simulink model "BMS_DCDC_Manager_V1"  (R2024b)
settings: Solver=FixedStepDiscrete  StartTime=0.0  StopTime=1  FixedStep=0.1  RelTol=1e-3
settings Model: Creator=Jingjing.jiang  LastModifiedBy=Jingjing.jiang
settings DataIOCC: SaveFormat=StructureWithTime

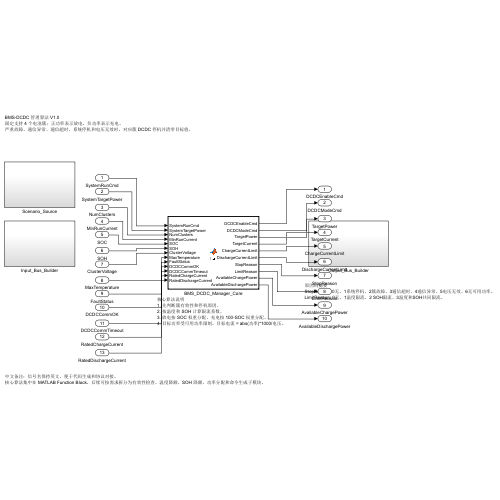
[thumbnail: Simulink's stored preview of the top-level diagram]
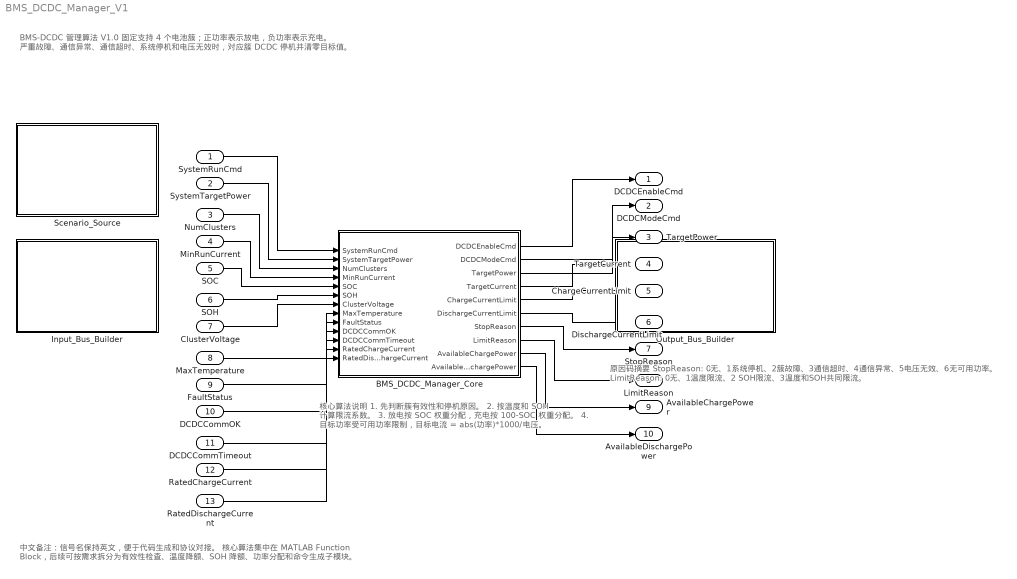
== system BMS_DCDC_Manager_V1 ==
  note: BMS-DCDC 管理算法 V1.0
      | 固定支持 4 个电池簇；正功率表示放电，负功率表示充电。
      | 严重故障、通信异常、通信超时、系统停机和电压无效时，对应簇 DCDC 停机并清零目标值。
  note: 中文备注：信号名保持英文，便于代码生成和协议对接。
      | 核心算法集中在 MATLAB Function Block，后续可按需求拆分为有效性检查、温度降额、SOH 降额、功率分配和命令生成子模块。
  note: 核心算法说明
      | 1. 先判断簇有效性和停机原因。
      | 2. 按温度和 SOH 计算限流系数。
      | 3. 放电按 SOC 权重分配，充电按 100-SOC 权重分配。
      | 4. 目标功率受可用功率限制，目标电流 = abs(功率)*1000/电压。
  note: 原因码摘要
      | StopReason: 0无、1系统停机、2簇故障、3通信超时、4通信异常、5电压无效、6无可用功率。
      | LimitReason: 0无、1温度限流、2 SOH限流、3温度和SOH共同限流。
  SystemRunCmd : Inport  OutDataTypeStr=boolean  PortDimensions=1
  SystemTargetPower : Inport  Port=2  OutDataTypeStr=double  PortDimensions=1
  NumClusters : Inport  Port=3  OutDataTypeStr=uint8  PortDimensions=1
  MinRunCurrent : Inport  Port=4  OutDataTypeStr=double  PortDimensions=1
  SOC : Inport  Port=5  OutDataTypeStr=double  PortDimensions=4
  SOH : Inport  Port=6  OutDataTypeStr=double  PortDimensions=4
  ClusterVoltage : Inport  Port=7  OutDataTypeStr=double  PortDimensions=4
  MaxTemperature : Inport  Port=8  OutDataTypeStr=double  PortDimensions=4
  FaultStatus : Inport  Port=9  OutDataTypeStr=boolean  PortDimensions=4
  DCDCCommOK : Inport  Port=10  OutDataTypeStr=boolean  PortDimensions=4
  DCDCCommTimeout : Inport  Port=11  OutDataTypeStr=boolean  PortDimensions=4
  RatedChargeCurrent : Inport  Port=12  OutDataTypeStr=double  PortDimensions=4
  RatedDischargeCurrent : Inport  Port=13  OutDataTypeStr=double  PortDimensions=4
  BMS_DCDC_Manager_Core : MATLAB Function  TreatAsAtomicUnit=on
  Input_Bus_Builder : Subsystem
  Output_Bus_Builder : Subsystem
  Scenario_Source : Subsystem
  DCDCEnableCmd : Outport  OutDataTypeStr=boolean  PortDimensions=4
  DCDCModeCmd : Outport  Port=2  OutDataTypeStr=uint8  PortDimensions=4
  TargetPower : Outport  Port=3  OutDataTypeStr=double  PortDimensions=4
  TargetCurrent : Outport  Port=4  OutDataTypeStr=double  PortDimensions=4
  ChargeCurrentLimit : Outport  Port=5  OutDataTypeStr=double  PortDimensions=4
  DischargeCurrentLimit : Outport  Port=6  OutDataTypeStr=double  PortDimensions=4
  StopReason : Outport  Port=7  OutDataTypeStr=uint16  PortDimensions=4
  LimitReason : Outport  Port=8  OutDataTypeStr=uint16  PortDimensions=4
  AvailableChargePower : Outport  Port=9  OutDataTypeStr=double  PortDimensions=4
  AvailableDischargePower : Outport  Port=10  OutDataTypeStr=double  PortDimensions=4
  wires:
  SystemRunCmd/1 -> BMS_DCDC_Manager_Core/1(SystemRunCmd)
  SystemTargetPower/1 -> BMS_DCDC_Manager_Core/2(SystemTargetPower)
  NumClusters/1 -> BMS_DCDC_Manager_Core/3(NumClusters)
  MinRunCurrent/1 -> BMS_DCDC_Manager_Core/4(MinRunCurrent)
  SOC/1 -> BMS_DCDC_Manager_Core/5(SOC)
  SOH/1 -> BMS_DCDC_Manager_Core/6(SOH)
  ClusterVoltage/1 -> BMS_DCDC_Manager_Core/7(ClusterVoltage)
  MaxTemperature/1 -> BMS_DCDC_Manager_Core/8(MaxTemperature)
  FaultStatus/1 -> BMS_DCDC_Manager_Core/9(FaultStatus)
  DCDCCommOK/1 -> BMS_DCDC_Manager_Core/10(DCDCCommOK)
  DCDCCommTimeout/1 -> BMS_DCDC_Manager_Core/11(DCDCCommTimeout)
  RatedChargeCurrent/1 -> BMS_DCDC_Manager_Core/12(RatedChargeCurrent)
  RatedDischargeCurrent/1 -> BMS_DCDC_Manager_Core/13(RatedDischargeCurrent)
  BMS_DCDC_Manager_Core/1(DCDCEnableCmd) -> DCDCEnableCmd/1
  BMS_DCDC_Manager_Core/2(DCDCModeCmd) -> DCDCModeCmd/1
  BMS_DCDC_Manager_Core/3(TargetPower) -> TargetPower/1
  BMS_DCDC_Manager_Core/4(TargetCurrent) -> TargetCurrent/1
  BMS_DCDC_Manager_Core/5(ChargeCurrentLimit) -> ChargeCurrentLimit/1
  BMS_DCDC_Manager_Core/6(DischargeCurrentLimit) -> DischargeCurrentLimit/1
  BMS_DCDC_Manager_Core/7(StopReason) -> StopReason/1
  BMS_DCDC_Manager_Core/8(LimitReason) -> LimitReason/1
  BMS_DCDC_Manager_Core/9(AvailableChargePower) -> AvailableChargePower/1
  BMS_DCDC_Manager_Core/10(AvailableDischargePower) -> AvailableDischargePower/1

== system BMS_DCDC_Manager_V1/Input_Bus_Builder ==
  note: 输入接口说明
      | 系统级输入：SystemRunCmd、SystemTargetPower、NumClusters、MinRunCurrent。
      | 簇级数组固定 4 维：SOC、SOH、电压、温度、故障、通信和额定电流。

== system BMS_DCDC_Manager_V1/Output_Bus_Builder ==
  note: 输出接口说明
      | DCDCEnableCmd：启停命令。
      | DCDCModeCmd：0=待机，1=充电，2=放电，3=故障。
      | TargetCurrent 始终为正值，方向由模式命令区分。

== system BMS_DCDC_Manager_V1/Scenario_Source ==
  note: 测试激励 / Scenario_Source
      | 默认场景数据来自 BMS_DCDC_Params.m。
      | TC01~TC08 可在自检脚本和后续测试模型中扩展。

== matlab function BMS_DCDC_Manager_V1/BMS_DCDC_Manager_Core ==
  data: SystemRunCmd input; DCDCEnableCmd output; SystemTargetPower input; NumClusters input; MinRunCurrent input; SOC input; SOH input; ClusterVoltage input; MaxTemperature input; FaultStatus input; DCDCCommOK input; DCDCCommTimeout input; RatedChargeCurrent input; RatedDischargeCurrent input; DCDCModeCmd output; TargetPower output; TargetCurrent output; ChargeCurrentLimit output; DischargeCurrentLimit output; StopReason output; LimitReason output; AvailableChargePower output; AvailableDischargePower output
function [DCDCEnableCmd, DCDCModeCmd, TargetPower, TargetCurrent, ...                                                             
                                                                                                                                     ChargeCurrentLimit, DischargeCurrentLimit, StopReason, LimitReason, ...                                                       
                                                                                                                                     AvailableChargePower, AvailableDischargePower] = fcn(SystemRunCmd, SystemTargetPower, NumClusters, MinRunCurrent, ...         
                                                                                                                                     SOC, SOH, ClusterVoltage, MaxTemperature, FaultStatus, DCDCCommOK, DCDCCommTimeout, RatedChargeCurrent, RatedDischargeCurrent)
                                                                                                                                 %#codegen                                                                                                                         
                                                                                                                                 % BMS-DCDC 管理算法 V1.0：调用根目录核心函数。                                                                                                   
                                                                                                                                 % 中文备注：模型固定 4 个簇，簇级输入输出均为 4 维数组。                                                                                                  
                                                                                                                                 [DCDCEnableCmd, DCDCModeCmd, TargetPower, TargetCurrent, ...                                                                      
                                                                                                                                     ChargeCurrentLimit, DischargeCurrentLimit, StopReason, LimitReason, ...                                                       
                                                                                                                                     AvailableChargePower, AvailableDischargePower] = ...                                                                          
                                                                                                                                     BMS_DCDC_Manager_Core(SystemRunCmd, SystemTargetPower, NumClusters, MinRunCurrent, ...                                        
                                                                                                                                     SOC, SOH, ClusterVoltage, MaxTemperature, FaultStatus, ...                                                                    
                                                                                                                                     DCDCCommOK, DCDCCommTimeout, RatedChargeCurrent, RatedDischargeCurrent);                                                      
                                                                                                                                 end
